simulink library "Hquad_control_LIB_LQRI"  (Simulink 7.6)
settings: Solver=ode45  StartTime=0.0  StopTime=10.0  RelTol=1e-3
values from neighbouring files (symbols this model uses):
  delay_pade_order = 0    [kostas_malakies.mat]    (also in kostas_malakies2.mat; main.m; main_last.m)
  g = 9.8065    [kostas_malakies.mat]    (also in kostas_malakies2.mat; load_PMModel.m = 9.81; main_last.m; matlab.mat)
  K_I_lqri_x = 0.330095898719    [kostas_malakies.mat]    (also in kostas_malakies2.mat)
  K_I_lqri_y = -0.330255855134    [kostas_malakies.mat]    (also in kostas_malakies2.mat)
  K_I_lqri_yaw = -0.366670548052    [kostas_malakies.mat]    (also in kostas_malakies2.mat)
  K_I_lqri_z = 0.689854163424    [kostas_malakies.mat]    (also in kostas_malakies2.mat)
  K_lqri_x = [-0.894732962063 -0.662437896475 0.0253750911961 0.0106501878726]    [kostas_malakies.mat]    (also in kostas_malakies2.mat)
  K_lqri_y = [0.897498772304 0.669088738193 0.0296050685235 0.0123545448922]    [kostas_malakies.mat]    (also in kostas_malakies2.mat)
  K_lqri_yaw = [1.88702639282 0.555643586179]    [kostas_malakies.mat]    (also in kostas_malakies2.mat)
  K_lqri_z = [-2.31070216446 -2.1452727372]    [kostas_malakies.mat]    (also in kostas_malakies2.mat)
  kalm_lqri_x =     [kostas_malakies.mat]    (also in kostas_malakies2.mat)
  kalm_lqri_y =     [kostas_malakies.mat]    (also in kostas_malakies2.mat)
  kalm_lqri_yaw =     [kostas_malakies.mat]    (also in kostas_malakies2.mat)
  kalm_lqri_z =     [kostas_malakies.mat]    (also in kostas_malakies2.mat)
  mass = 0.66    [kostas_malakies.mat]    (also in kostas_malakies2.mat; load_PMModel.m = 0.687; main_last.m)
  MAX_ANGLE = 0.261799387799    [kostas_malakies.mat]    (also in kostas_malakies2.mat; main.m; main_last.m)
  MAX_FORCE = 2    [kostas_malakies.mat]    (also in kostas_malakies2.mat; main.m; main_last.m)
  MAX_YAW_RATE = 3.14159265359    [kostas_malakies.mat]    (also in kostas_malakies2.mat; main.m; main_last.m)
  Ts = 0.02    [kostas_malakies.mat]    (also in kostas_malakies2.mat; main.m; main_last.m; matlab.mat = 0.08)
undefined symbols (not defined in the file or in its folder): DiscIntNeverNeededParam
libraries: Hquad_control_LIB_LQRI x17, simulink x9
settings Model: Creator=andi  LastModifiedBy=burrimi

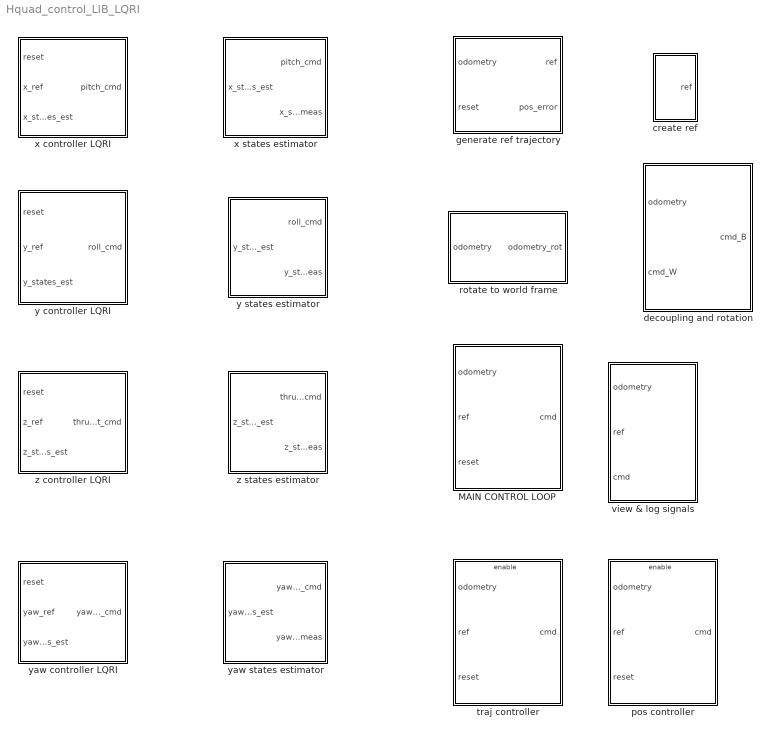
== system Hquad_control_LIB_LQRI ==
  MAIN CONTROL LOOP : Subsystem  TreatAsAtomicUnit=on
  create ref : Subsystem
  decoupling and rotation : Subsystem  Priority=3  TreatAsAtomicUnit=on
  generate ref trajectory : Subsystem
  pos controller : Subsystem
  rotate to world frame : Subsystem  Priority=1
  traj controller : Subsystem
  view & log signals : Subsystem
  "x controller LQRI  " : Subsystem
  x states estimator : Subsystem
  y controller LQRI : Subsystem
  y states estimator : Subsystem
  yaw controller LQRI : Subsystem
  yaw states estimator : Subsystem
  z controller LQRI : Subsystem
  z states estimator : Subsystem

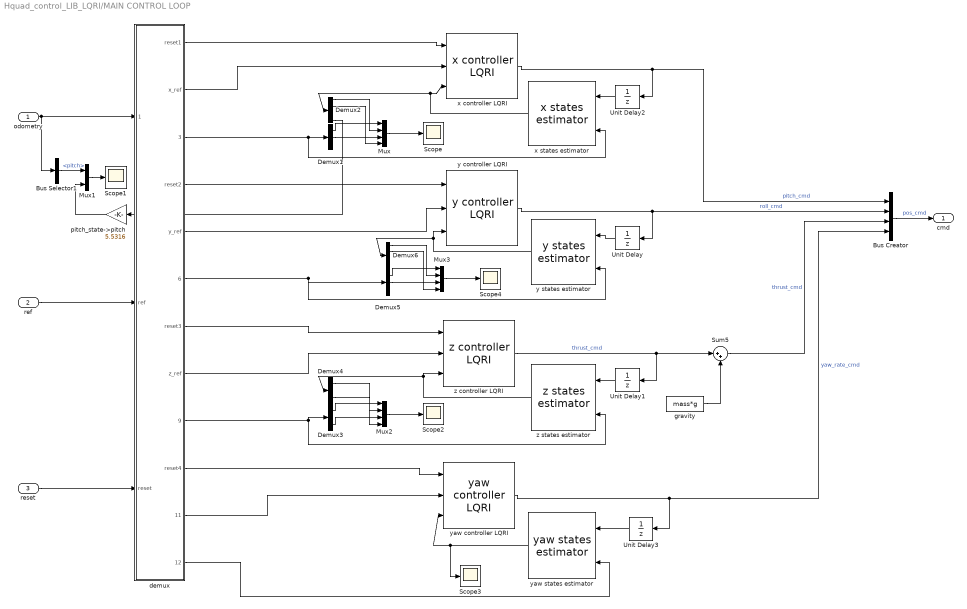
== system Hquad_control_LIB_LQRI/MAIN CONTROL LOOP ==
  odometry : Inport
  ref : Inport  Port=2
  reset : Inport  Port=3
  Bus Creator : BusCreator
  Bus Selector1 : BusSelector  OutputSignals=rpy.pitch
  Demux1 : Demux  Outputs=3
  Demux2 : Demux
  Demux3 : Demux  Outputs=2
  Demux4 : Demux  Outputs=2
  Demux5 : Demux  Outputs=3
  Demux6 : Demux
  Mux : Mux
  Mux1 : Mux  Inputs=2
  Mux2 : Mux
  Mux3 : Mux
  Scope{,1..4} (5 alike) : Scope
      Scope settings: TimeRange=8.564360869565219  YMin=-0.05  YMax=1.05  SaveName=ScopeData13
      Scope1 settings: YMin=-0.4  YMax=1.4  SaveName=ScopeData14
      Scope2 settings: YMin=-0.4  YMax=1.4  SaveName=ScopeData15
      Scope3 settings: YMin=-0.4  YMax=1.4  SaveName=ScopeData16
      Scope4 settings: TimeRange=8.564360869565219  YMin=-0.05  YMax=1.05  SaveName=ScopeData4
  Sum5 : Sum  Inputs=|++
  Unit Delay{,1..3} (4 alike) : UnitDelay  SampleTime=Ts
  demux : Subsystem
  gravity : Constant  Value=mass*g
  pitch_state->pitch : Gain  Gain=5.5316
  "x controller LQRI  " : Hquad_control_LIB_LQRI/x controller LQRI    SystemSampleTime=-1
  x states estimator : Hquad_control_LIB_LQRI/x states estimator  SystemSampleTime=-1
  y controller LQRI : Hquad_control_LIB_LQRI/y controller LQRI  SystemSampleTime=-1
  y states estimator : Hquad_control_LIB_LQRI/y states estimator  SystemSampleTime=-1
  yaw controller LQRI : Hquad_control_LIB_LQRI/yaw controller LQRI  SystemSampleTime=-1
  yaw states estimator : Hquad_control_LIB_LQRI/yaw states estimator  SystemSampleTime=-1
  z controller LQRI : Hquad_control_LIB_LQRI/z controller LQRI  SystemSampleTime=-1
  z states estimator : Hquad_control_LIB_LQRI/z states estimator  SystemSampleTime=-1
  cmd : Outport
  wires:
  demux/7(reset3) -> z controller LQRI/1
  demux/8(z_ref) -> z controller LQRI/2
  Demux4/2 -> Mux2/4
  Demux6/2 -> Mux3/4
  Demux5/2 -> Mux3/3
  Demux6/1 -> Mux3/2
  Demux5/1 -> Mux3/1
  Mux3/1 -> Scope4/1
  demux/4(reset2) -> y controller LQRI/1
  demux/5(y_ref) -> y controller LQRI/2
  gravity/1 -> Sum5/2
  yaw states estimator/1 -> Scope3/1, yaw controller LQRI/3
  z controller LQRI/1 -> Sum5/1, Unit Delay1/1  "thrust_cmd"
  Demux3/2 -> Mux2/3
  Demux4/1 -> Mux2/2
  Demux3/1 -> Mux2/1
  Mux2/1 -> Scope2/1
  pitch_state->pitch/1 -> Mux1/2
  Demux2/4 -> pitch_state->pitch/1
  Bus Selector1/1 -> Mux1/1  "<pitch>"
  Mux1/1 -> Scope1/1
  Demux2/2 -> Mux/4
  Demux1/2 -> Mux/3
  Demux2/1 -> Mux/2
  Demux1/1 -> Mux/1
  Mux/1 -> Scope/1
  z states estimator/1 -> Demux4/1, z controller LQRI/3
  y controller LQRI/1 -> Bus Creator/2, Unit Delay/1  "roll_cmd"
  "x controller LQRI  "/1 -> Bus Creator/1, Unit Delay2/1  "pitch_cmd"
  y states estimator/1 -> Demux6/1, y controller LQRI/3
  x states estimator/1 -> Demux2/1, "x controller LQRI  "/3
  demux/2(x_ref) -> "x controller LQRI  "/2
  Unit Delay/1 -> y states estimator/1
  Unit Delay1/1 -> z states estimator/1
  Unit Delay2/1 -> x states estimator/1
  demux/12(yaw_states_meas) -> yaw states estimator/2
  yaw controller LQRI/1 -> Bus Creator/4, Unit Delay3/1  "yaw_rate_cmd"
  odometry/1 -> Bus Selector1/1, demux/1(odometry)
  ref/1 -> demux/2(ref)
  reset/1 -> demux/3(reset)
  demux/1(reset1) -> "x controller LQRI  "/1
  demux/10(reset4) -> yaw controller LQRI/1
  Bus Creator/1 -> cmd/1  "pos_cmd"
  demux/3(x_states_meas) -> Demux1/1, x states estimator/2
  demux/6(y_states_meas) -> Demux5/1, y states estimator/2
  demux/9(z_states_meas) -> Demux3/1, z states estimator/2
  demux/11(yaw_ref) -> yaw controller LQRI/2
  Sum5/1 -> Bus Creator/3  "thrust_cmd"
  Unit Delay3/1 -> yaw states estimator/1

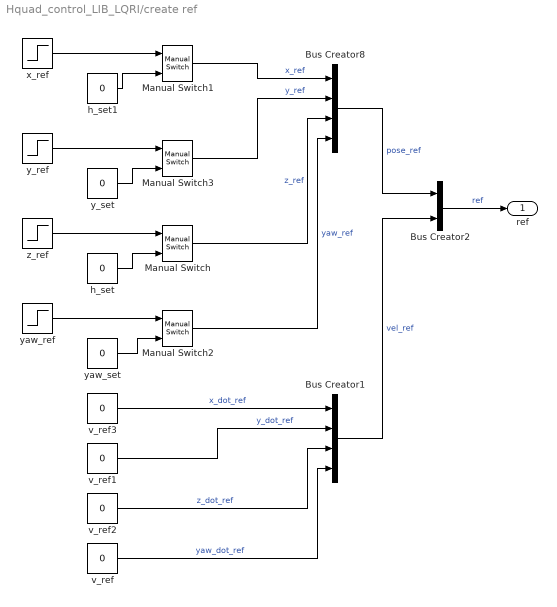
== system Hquad_control_LIB_LQRI/create ref ==
  Bus Creator1 : BusCreator
  Bus Creator2 : BusCreator  Inputs=2
  Bus Creator8 : BusCreator
  Manual Switch{,1..3} (4 alike) : simulink/Signal Routing/Manual Switch  SystemSampleTime=-1  sw=1  action=0  varsize=off
  h_set : Constant  Value=0  OutDataTypeStr=double  SampleTime=-1
  h_set1 : Constant  Value=0  OutDataTypeStr=double  SampleTime=-1
  v_ref{,1..3} (4 alike) : Constant  Value=0  OutDataTypeStr=double  SampleTime=-1
  x_ref : Step  Time=5  SampleTime=0
  y_ref : Step  Time=15  SampleTime=0
  y_set : Constant  Value=0  OutDataTypeStr=double  SampleTime=-1
  yaw_ref : Step  Time=20  After=pi  SampleTime=0
  "yaw_set  " : Constant  Value=0  OutDataTypeStr=double  SampleTime=-1
  z_ref : Step  Time=15  SampleTime=0
  ref : Outport
  wires:
  yaw_ref/1 -> Manual Switch2/1
  "yaw_set  "/1 -> Manual Switch2/2
  h_set/1 -> Manual Switch/2
  z_ref/1 -> Manual Switch/1
  y_ref/1 -> Manual Switch3/1
  y_set/1 -> Manual Switch3/2
  h_set1/1 -> Manual Switch1/2
  Bus Creator2/1 -> ref/1  "ref"
  Bus Creator8/1 -> Bus Creator2/1  "pose_ref"
  Bus Creator1/1 -> Bus Creator2/2  "vel_ref"
  Manual Switch1/1 -> Bus Creator8/1  "x_ref"
  Manual Switch3/1 -> Bus Creator8/2  "y_ref"
  Manual Switch2/1 -> Bus Creator8/4  "yaw_ref"
  Manual Switch/1 -> Bus Creator8/3  "z_ref"
  v_ref/1 -> Bus Creator1/4  "yaw_dot_ref"
  v_ref3/1 -> Bus Creator1/1  "x_dot_ref"
  v_ref1/1 -> Bus Creator1/2  "y_dot_ref"
  v_ref2/1 -> Bus Creator1/3  "z_dot_ref"
  x_ref/1 -> Manual Switch1/1

== system Hquad_control_LIB_LQRI/decoupling and rotation ==
  note: 
  odometry : Inport
  cmd_W : Inport  Port=2
  Bus Selector1 : BusSelector  OutputSignals=rpy.yaw
  Bus Selector2 : BusSelector  OutputSignals=rpy.roll,rpy.pitch
  "decoupling " : Subsystem
  rotate_to_quat_frame : Subsystem
  cmd_B : Outport
  wires:
  Bus Selector2/2 -> "decoupling "/2("pitch_meas  ")  "<pitch>"
  Bus Selector2/1 -> "decoupling "/1("roll_meas  ")  "<roll>"
  cmd_W/1 -> "decoupling "/3(cmd)
  Bus Selector1/1 -> rotate_to_quat_frame/1(yaw_meas)  "<yaw>"
  odometry/1 -> Bus Selector2/1, Bus Selector1/1
  "decoupling "/1("cmd_comp  ") -> rotate_to_quat_frame/2(cmd_comp)  "cmd_comp"
  rotate_to_quat_frame/1("cmd_rot  ") -> cmd_B/1  "roll_cmd"

== system Hquad_control_LIB_LQRI/generate ref trajectory ==
  odometry : Inport
  reset : Inport  Port=2
  Bus Creator : BusCreator
  Bus Creator1 : BusCreator
  Bus Creator2 : BusCreator  Inputs=2
  Bus Selector : BusSelector  OutputSignals=pos,vel
  Demux : Demux  Outputs=2
  Demux1 : Demux  Outputs=3
  Demux2 : Demux  Outputs=3
  Embedded MATLAB Function : Stateflow chart  TreatAsAtomicUnit=on
  Unit Delay Resettable : simulink/Additional Math & Discrete/Additional Discrete/Unit Delay Resettable  SystemSampleTime=-1  vinit=0.0  tsamp=-1
  ref : Outport
  pos_error : Outport  Port=2
  wires:
  Bus Creator2/1 -> ref/1  "ref"
  reset/1 -> Unit Delay Resettable/2
  Bus Creator1/1 -> Bus Creator2/2  "vel_ref"
  Bus Creator/1 -> Bus Creator2/1  "pose_ref"
  Demux/2 -> Bus Creator1/4  "yaw_dot_ref"
  Demux2/3 -> Bus Creator1/3  "z_dot_ref"
  Demux2/2 -> Bus Creator1/2  "y_dot_ref"
  Demux2/1 -> Bus Creator1/1  "x_dot_ref"
  Demux/1 -> Bus Creator/4  "yaw_ref"
  Demux1/3 -> Bus Creator/3  "z_ref"
  Demux1/2 -> Bus Creator/2  "y_ref"
  Demux1/1 -> Bus Creator/1  "x_ref"
  Embedded MATLAB Function/2(vel_ref) -> Demux2/1
  Embedded MATLAB Function/1(pos_ref) -> Demux1/1
  Embedded MATLAB Function/4(error) -> pos_error/1  "pos_error"
  Embedded MATLAB Function/3(yaw_ref) -> Demux/1
  Embedded MATLAB Function/5(waypoint_id_out) -> Unit Delay Resettable/1
  Unit Delay Resettable/1 -> Embedded MATLAB Function/3(waypoint_id)
  odometry/1 -> Bus Selector/1
  Bus Selector/1 -> Embedded MATLAB Function/1(pos)  "<pos>"
  Bus Selector/2 -> Embedded MATLAB Function/2(vel)  "<vel>"

== system Hquad_control_LIB_LQRI/pos controller ==
  odometry : Inport
  ref : Inport  Port=2
  reset : Inport  Port=3
  Enable : EnablePort  StatesWhenEnabling=reset
  MAIN CONTROL LOOP : Hquad_control_LIB_LQRI/MAIN CONTROL LOOP  SystemSampleTime=-1
  decoupling and rotation : Hquad_control_LIB_LQRI/decoupling and rotation  Priority=3  SystemSampleTime=-1
  rotate to world frame : Hquad_control_LIB_LQRI/rotate to world frame  Priority=1  SystemSampleTime=-1
  view & log signals : Hquad_control_LIB_LQRI/view & log signals  SystemSampleTime=-1
  cmd : Outport
  wires:
  ref/1 -> MAIN CONTROL LOOP/2, view & log signals/2
  reset/1 -> MAIN CONTROL LOOP/3
  odometry/1 -> rotate to world frame/1
  rotate to world frame/1 -> view & log signals/1, decoupling and rotation/1, MAIN CONTROL LOOP/1
  MAIN CONTROL LOOP/1 -> view & log signals/3, decoupling and rotation/2
  decoupling and rotation/1 -> cmd/1

== system Hquad_control_LIB_LQRI/rotate to world frame ==
  odometry : Inport
  Bus Creator1 : BusCreator  Inputs=3
  Bus Creator5 : BusCreator
  Bus Selector1 : BusSelector  OutputSignals=rpy.roll,rpy.pitch
  Bus Selector2 : BusSelector  OutputSignals=ang_vel
  Bus Selector3 : BusSelector  OutputSignals=rpy.yaw
  Bus Selector6 : BusSelector  OutputSignals=pos,vel
  Embedded MATLAB Function : Stateflow chart  TreatAsAtomicUnit=on
  odometry_rot : Outport
  wires:
  Bus Selector1/2 -> Embedded MATLAB Function/2(pitch)  "<pitch>"
  Bus Selector1/1 -> Embedded MATLAB Function/1(roll)  "<roll>"
  Embedded MATLAB Function/2(pitch_rot) -> Bus Creator1/2  "pitch"
  Embedded MATLAB Function/1(roll_rot) -> Bus Creator1/1  "roll"
  Bus Creator1/1 -> Bus Creator5/3  "rpy"
  Bus Selector2/1 -> Bus Creator5/4  "<ang_vel>"
  odometry/1 -> Bus Selector2/1, Bus Selector6/1, Bus Selector1/1, Bus Selector3/1
  Bus Selector3/1 -> Bus Creator1/3, Embedded MATLAB Function/3(yaw)  "<yaw>"
  Bus Creator5/1 -> odometry_rot/1  "odom"
  Bus Selector6/1 -> Bus Creator5/1  "<pos>"
  Bus Selector6/2 -> Bus Creator5/2  "<vel>"

== system Hquad_control_LIB_LQRI/traj controller ==
  odometry : Inport
  ref : Inport  Port=2
  reset : Inport  Port=3
  Enable : EnablePort  StatesWhenEnabling=reset
  MAIN CONTROL LOOP : Hquad_control_LIB_LQRI/MAIN CONTROL LOOP  SystemSampleTime=-1
  Terminator : Terminator
  decoupling and rotation : Hquad_control_LIB_LQRI/decoupling and rotation  Priority=3  SystemSampleTime=-1
  generate ref trajectory : Hquad_control_LIB_LQRI/generate ref trajectory  SystemSampleTime=-1
  rotate to world frame : Hquad_control_LIB_LQRI/rotate to world frame  Priority=1  SystemSampleTime=-1
  view & log signals : Hquad_control_LIB_LQRI/view & log signals  SystemSampleTime=-1
  cmd : Outport
  wires:
  decoupling and rotation/1 -> cmd/1
  MAIN CONTROL LOOP/1 -> decoupling and rotation/2, view & log signals/3
  rotate to world frame/1 -> MAIN CONTROL LOOP/1, decoupling and rotation/1, view & log signals/1
  odometry/1 -> rotate to world frame/1, generate ref trajectory/1
  ref/1 -> Terminator/1
  reset/1 -> MAIN CONTROL LOOP/3, generate ref trajectory/2
  generate ref trajectory/1 -> view & log signals/2, MAIN CONTROL LOOP/2

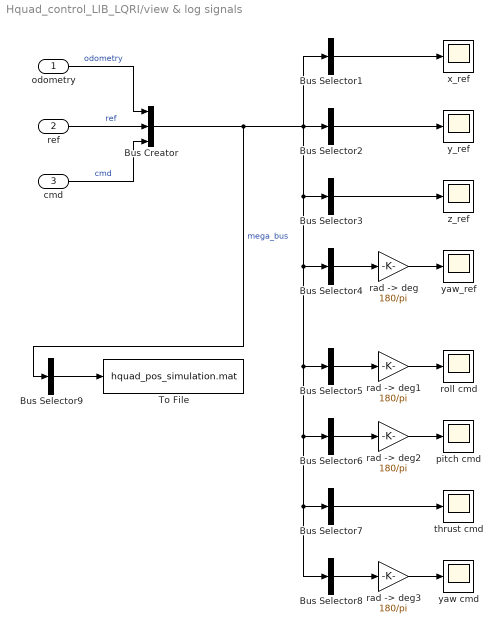
== system Hquad_control_LIB_LQRI/view & log signals ==
  odometry : Inport
  ref : Inport  Port=2
  cmd : Inport  Port=3
  Bus Creator : BusCreator  Inputs=3
  Bus Selector1 : BusSelector  OutputSignals=odometry.pos.x,odometry.vel.x_dot,ref.pose_ref.x_ref,ref.vel_ref.x_dot_ref  OutputAsBus=on
  Bus Selector2 : BusSelector  OutputSignals=odometry.pos.y,odometry.vel.y_dot,ref.pose_ref.y_ref,ref.vel_ref.y_dot_ref  OutputAsBus=on
  Bus Selector3 : BusSelector  OutputSignals=odometry.pos.z,odometry.vel.z_dot,ref.pose_ref.z_ref,ref.vel_ref.z_dot_ref  OutputAsBus=on
  Bus Selector4 : BusSelector  OutputSignals=odometry.rpy.yaw,odometry.ang_vel.ang_vel_z,ref.pose_ref.yaw_ref,ref.vel_ref.yaw_dot_ref  OutputAsBus=on
  Bus Selector5 : BusSelector  OutputSignals=odometry.rpy.roll,odometry.ang_vel.ang_vel_x,cmd.roll_cmd  OutputAsBus=on
  Bus Selector6 : BusSelector  OutputSignals=odometry.rpy.pitch,odometry.ang_vel.ang_vel_y,cmd.pitch_cmd  OutputAsBus=on
  Bus Selector7 : BusSelector  OutputSignals=odometry.pos.z,ref.pose_ref.z_ref,cmd.thrust_cmd  OutputAsBus=on
  Bus Selector8 : BusSelector  OutputSignals=odometry.rpy.yaw,odometry.ang_vel.ang_vel_z,cmd.yaw_rate_cmd  OutputAsBus=on
  Bus Selector9 : BusSelector  OutputSignals=odometry.pos.x,odometry.vel.x_dot,odometry.rpy.pitch,ref.pose_ref.x_ref,cmd.pitch_cmd,odometry.pos.y,odometry.vel.y_dot,odometry.rpy.roll,ref.pose_ref.y_ref,cmd.roll_cmd,odometry.pos.z,odometry.vel.z_dot,ref.pose_ref.z_ref,cmd.thrust_cmd,odometry.rpy.yaw,odometry.ang_vel.ang_vel_z,ref.pose_ref.yaw_ref,cmd.yaw_rate_cmd  OutputAsBus=on
  To File : ToFile  Filename=hquad_pos_simulation.mat  MatrixName=hquad_pos_simulation
  pitch cmd : Scope
      settings: YMin=-15  YMax=15  SaveName=ScopeData2
  rad -> deg{,1..3} (4 alike) : Gain  Gain=180/pi
  roll cmd : Scope
      settings: YMin=-100  YMax=100
  thrust cmd : Scope
      settings: YMin=-3  YMax=3  SaveName=ScopeData11
  x_ref : Scope
      settings: TimeRange=40  YMin=-1.5  YMax=1.5  SaveName=ScopeData3
  y_ref : Scope
      settings: TimeRange=40  YMin=-1.5  YMax=1.5
  yaw cmd : Scope
      settings: YMin=-60  YMax=-0  SaveName=ScopeData10
  yaw_ref : Scope
      settings: TimeRange=39.996  YMin=0  YMax=3250  SaveName=ScopeData8
  z_ref : Scope
      settings: YMin=-0.05  YMax=1.05  SaveName=ScopeData5
  wires:
  Bus Selector8/1 -> "rad -> deg3"/1
  Bus Selector6/1 -> "rad -> deg2"/1
  Bus Selector5/1 -> "rad -> deg1"/1
  Bus Selector7/1 -> thrust cmd/1
  Bus Selector4/1 -> "rad -> deg"/1
  Bus Selector3/1 -> z_ref/1
  Bus Selector2/1 -> y_ref/1
  Bus Selector1/1 -> x_ref/1
  Bus Creator/1 -> Bus Selector8/1, Bus Selector7/1, Bus Selector6/1, Bus Selector5/1, Bus Selector4/1, Bus Selector3/1, Bus Selector2/1, Bus Selector1/1, Bus Selector9/1  "mega_bus"
  cmd/1 -> Bus Creator/3  "cmd"
  ref/1 -> Bus Creator/2  "ref"
  odometry/1 -> Bus Creator/1  "odometry"
  "rad -> deg3"/1 -> yaw cmd/1
  "rad -> deg2"/1 -> pitch cmd/1
  "rad -> deg1"/1 -> roll cmd/1
  "rad -> deg"/1 -> yaw_ref/1
  Bus Selector9/1 -> To File/1

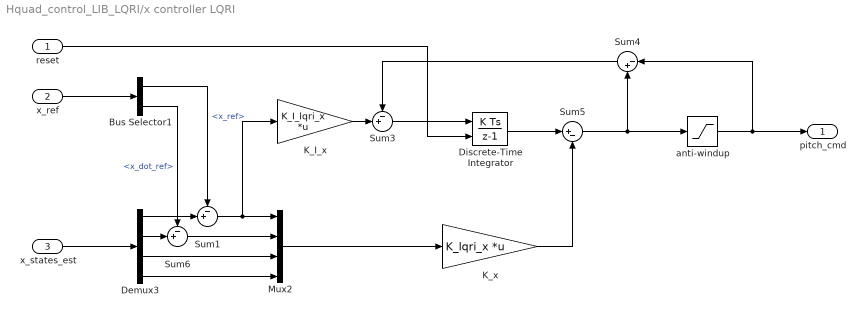
== system Hquad_control_LIB_LQRI/x controller LQRI   ==
  reset : Inport  PortDimensions=1
  "x_ref  " : Inport  Port=2  PortDimensions=2
  "x_states_est  " : Inport  Port=3
  Bus Selector1 : BusSelector  OutputSignals=x_ref,x_dot_ref
  Demux3 : Demux
  Discrete-Time Integrator : DiscreteIntegrator  ExternalReset=rising  SampleTime=Ts  ICPrevOutput=DiscIntNeverNeededParam  ICPrevScaledInput=DiscIntNeverNeededParam
  K_I_x : Gain  Gain=K_I_lqri_x  Multiplication=Matrix(K*u)  OutDataTypeStr=single
  K_x : Gain  Gain=K_lqri_x  Multiplication=Matrix(K*u)
  Mux2 : Mux
  Sum1 : Sum  Inputs=-+|
  Sum3 : Sum  Inputs=-+|
  Sum4 : Sum  Inputs=|-+
  Sum5 : Sum  Inputs=|+-
  Sum6 : Sum  Inputs=-+|
  anti-windup : Saturate  UpperLimit=MAX_ANGLE  LowerLimit=-MAX_ANGLE
  "pitch_cmd   " : Outport  PortDimensions=1
  wires:
  Demux3/2 -> Sum6/2
  Bus Selector1/2 -> Sum6/1  "<x_dot_ref>"
  Bus Selector1/1 -> Sum1/1  "<x_ref>"
  Sum6/1 -> Mux2/2
  "x_ref  "/1 -> Bus Selector1/1
  Sum3/1 -> Discrete-Time Integrator/1
  Sum4/1 -> Sum3/1
  Discrete-Time Integrator/1 -> Sum5/1
  K_x/1 -> Sum5/2
  anti-windup/1 -> "pitch_cmd   "/1, Sum4/1
  reset/1 -> Discrete-Time Integrator/2
  "x_states_est  "/1 -> Demux3/1
  Mux2/1 -> K_x/1
  Demux3/1 -> Sum1/2
  Sum1/1 -> Mux2/1, K_I_x/1
  Demux3/3 -> Mux2/3
  Demux3/4 -> Mux2/4
  K_I_x/1 -> Sum3/2
  Sum5/1 -> anti-windup/1, Sum4/2

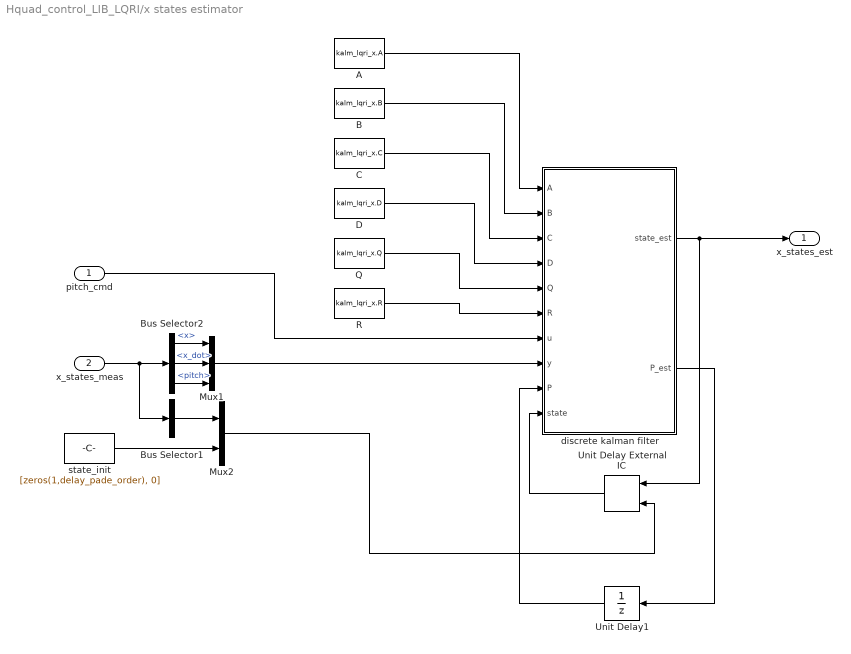
== system Hquad_control_LIB_LQRI/x states estimator ==
  pitch_cmd : Inport  PortDimensions=1
  x_states_meas : Inport  Port=2  PortDimensions=3
  A : Constant  Value=kalm_lqri_x.A
  B : Constant  Value=kalm_lqri_x.B
  Bus Selector1 : BusSelector  OutputSignals=x,x_dot,pitch  OutputAsBus=on
  Bus Selector2 : BusSelector  OutputSignals=x,x_dot,pitch
  C : Constant  Value=kalm_lqri_x.C
  D : Constant  Value=kalm_lqri_x.D
  Mux1 : Mux  Inputs=3
  Mux2 : Mux  Inputs=2
  Q : Constant  Value=kalm_lqri_x.Q
  R : Constant  Value=kalm_lqri_x.R
  Unit Delay External IC : simulink/Additional Math & Discrete/Additional Discrete/Unit Delay External IC  SystemSampleTime=-1  tsamp=-1
  Unit Delay1 : UnitDelay  X0=kalm_lqri_x.Z  SampleTime=Ts
  discrete kalman filter : Stateflow chart  TreatAsAtomicUnit=on
  state_init : Constant  Value=[zeros(1,delay_pade_order), 0]
  x_states_est : Outport  PortDimensions=4+delay_pade_order
  wires:
  x_states_meas/1 -> Bus Selector1/1, Bus Selector2/1
  state_init/1 -> Mux2/2
  Bus Selector1/1 -> Mux2/1
  A/1 -> discrete kalman filter/1(A)
  B/1 -> discrete kalman filter/2(B)
  C/1 -> discrete kalman filter/3(C)
  D/1 -> discrete kalman filter/4(D)
  discrete kalman filter/1(state_est) -> x_states_est/1, Unit Delay External IC/1
  Unit Delay External IC/1 -> discrete kalman filter/10(state)
  discrete kalman filter/2(P_est) -> Unit Delay1/1
  Unit Delay1/1 -> discrete kalman filter/9(P)
  Mux2/1 -> Unit Delay External IC/2
  pitch_cmd/1 -> discrete kalman filter/7(u)
  Bus Selector2/1 -> Mux1/1  "<x>"
  Bus Selector2/2 -> Mux1/2  "<x_dot>"
  Bus Selector2/3 -> Mux1/3  "<pitch>"
  Mux1/1 -> discrete kalman filter/8(y)
  Q/1 -> discrete kalman filter/5(Q)
  R/1 -> discrete kalman filter/6(R)

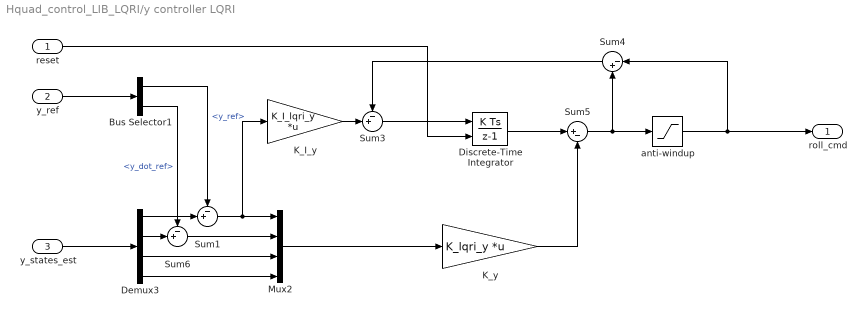
== system Hquad_control_LIB_LQRI/y controller LQRI ==
  reset : Inport  PortDimensions=1
  "y_ref  " : Inport  Port=2  PortDimensions=2
  "y_states_est  " : Inport  Port=3
  Bus Selector1 : BusSelector  OutputSignals=y_ref,y_dot_ref
  Demux3 : Demux
  Discrete-Time Integrator : DiscreteIntegrator  ExternalReset=rising  SampleTime=Ts  ICPrevOutput=DiscIntNeverNeededParam  ICPrevScaledInput=DiscIntNeverNeededParam
  K_I_y : Gain  Gain=K_I_lqri_y  Multiplication=Matrix(K*u)  OutDataTypeStr=single
  K_y : Gain  Gain=K_lqri_y  Multiplication=Matrix(K*u)
  Mux2 : Mux
  Sum1 : Sum  Inputs=-+|
  Sum3 : Sum  Inputs=-+|
  Sum4 : Sum  Inputs=|-+
  Sum5 : Sum  Inputs=|+-
  Sum6 : Sum  Inputs=-+|
  anti-windup : Saturate  UpperLimit=MAX_ANGLE  LowerLimit=-MAX_ANGLE
  "roll_cmd   " : Outport  PortDimensions=1
  wires:
  Demux3/2 -> Sum6/2
  Bus Selector1/2 -> Sum6/1  "<y_dot_ref>"
  Bus Selector1/1 -> Sum1/1  "<y_ref>"
  Sum6/1 -> Mux2/2
  "y_ref  "/1 -> Bus Selector1/1
  Sum3/1 -> Discrete-Time Integrator/1
  Sum4/1 -> Sum3/1
  Discrete-Time Integrator/1 -> Sum5/1
  K_y/1 -> Sum5/2
  anti-windup/1 -> "roll_cmd   "/1, Sum4/1
  reset/1 -> Discrete-Time Integrator/2
  "y_states_est  "/1 -> Demux3/1
  Mux2/1 -> K_y/1
  Demux3/1 -> Sum1/2
  Sum1/1 -> Mux2/1, K_I_y/1
  Demux3/3 -> Mux2/3
  Demux3/4 -> Mux2/4
  K_I_y/1 -> Sum3/2
  Sum5/1 -> anti-windup/1, Sum4/2

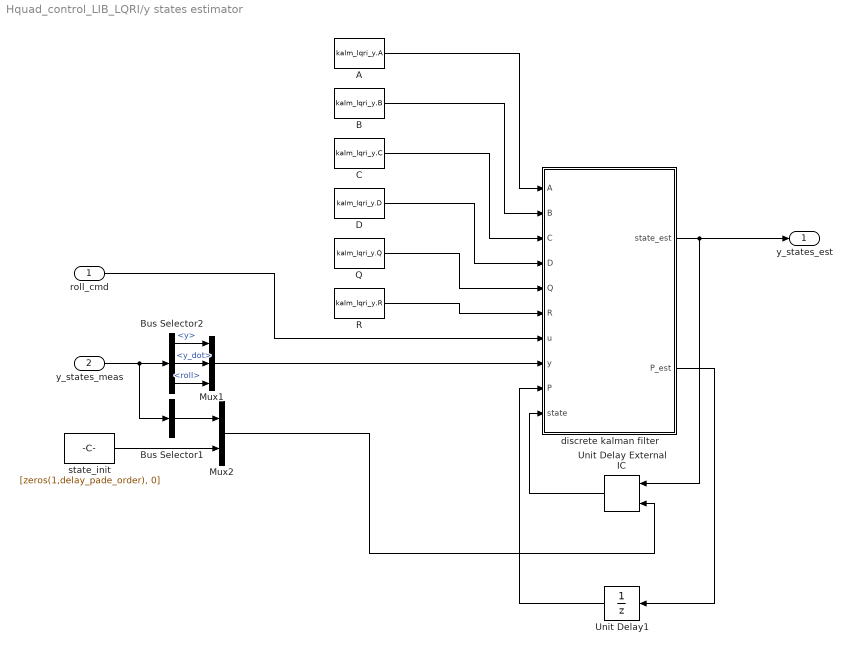
== system Hquad_control_LIB_LQRI/y states estimator ==
  roll_cmd : Inport  PortDimensions=1
  y_states_meas : Inport  Port=2  PortDimensions=3
  A : Constant  Value=kalm_lqri_y.A
  B : Constant  Value=kalm_lqri_y.B
  Bus Selector1 : BusSelector  OutputSignals=y,y_dot,roll  OutputAsBus=on
  Bus Selector2 : BusSelector  OutputSignals=y,y_dot,roll
  C : Constant  Value=kalm_lqri_y.C
  D : Constant  Value=kalm_lqri_y.D
  Mux1 : Mux  Inputs=3
  Mux2 : Mux  Inputs=2
  Q : Constant  Value=kalm_lqri_y.Q
  R : Constant  Value=kalm_lqri_y.R
  Unit Delay External IC : simulink/Additional Math & Discrete/Additional Discrete/Unit Delay External IC  SystemSampleTime=-1  tsamp=-1
  Unit Delay1 : UnitDelay  X0=kalm_lqri_y.Z  SampleTime=Ts
  discrete kalman filter : Stateflow chart  TreatAsAtomicUnit=on
  state_init : Constant  Value=[zeros(1,delay_pade_order), 0]
  y_states_est : Outport  PortDimensions=4+delay_pade_order
  wires:
  y_states_meas/1 -> Bus Selector1/1, Bus Selector2/1
  state_init/1 -> Mux2/2
  Bus Selector1/1 -> Mux2/1
  A/1 -> discrete kalman filter/1(A)
  B/1 -> discrete kalman filter/2(B)
  C/1 -> discrete kalman filter/3(C)
  D/1 -> discrete kalman filter/4(D)
  discrete kalman filter/1(state_est) -> y_states_est/1, Unit Delay External IC/1
  Unit Delay External IC/1 -> discrete kalman filter/10(state)
  discrete kalman filter/2(P_est) -> Unit Delay1/1
  Unit Delay1/1 -> discrete kalman filter/9(P)
  Mux2/1 -> Unit Delay External IC/2
  roll_cmd/1 -> discrete kalman filter/7(u)
  Bus Selector2/1 -> Mux1/1  "<y>"
  Bus Selector2/2 -> Mux1/2  "<y_dot>"
  Bus Selector2/3 -> Mux1/3  "<roll>"
  Mux1/1 -> discrete kalman filter/8(y)
  Q/1 -> discrete kalman filter/5(Q)
  R/1 -> discrete kalman filter/6(R)

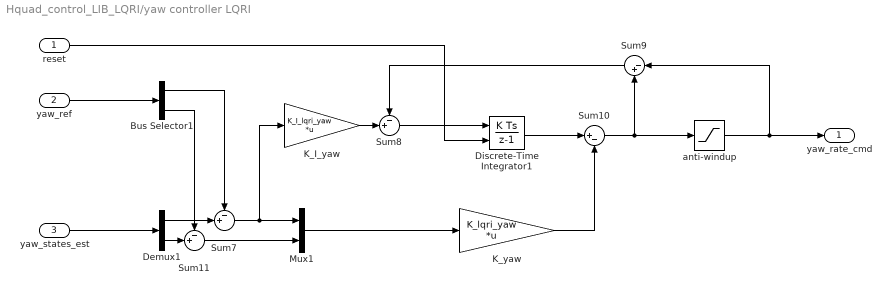
== system Hquad_control_LIB_LQRI/yaw controller LQRI ==
  reset : Inport  PortDimensions=1
  "yaw_ref  " : Inport  Port=2  PortDimensions=2
  "yaw_states_est  " : Inport  Port=3
  Bus Selector1 : BusSelector  OutputSignals=yaw_ref,yaw_dot_ref
  Demux1 : Demux  Outputs=2
  Discrete-Time Integrator1 : DiscreteIntegrator  ExternalReset=rising  SampleTime=Ts  ICPrevOutput=DiscIntNeverNeededParam  ICPrevScaledInput=DiscIntNeverNeededParam
  K_I_yaw : Gain  Gain=K_I_lqri_yaw  Multiplication=Matrix(K*u)  OutDataTypeStr=single
  K_yaw : Gain  Gain=K_lqri_yaw  Multiplication=Matrix(K*u)
  Mux1 : Mux  Inputs=2
  Sum10 : Sum  Inputs=|+-
  Sum11 : Sum  Inputs=-+|
  Sum7 : Sum  Inputs=-+|
  Sum8 : Sum  Inputs=-+|
  Sum9 : Sum  Inputs=|-+
  anti-windup : Saturate  UpperLimit=MAX_YAW_RATE  LowerLimit=-MAX_YAW_RATE
  "yaw_rate_cmd  " : Outport  PortDimensions=1
  wires:
  Demux1/2 -> Sum11/2
  Bus Selector1/2 -> Sum11/1
  Bus Selector1/1 -> Sum7/1
  Sum11/1 -> Mux1/2
  Sum8/1 -> Discrete-Time Integrator1/1
  Sum9/1 -> Sum8/1
  Discrete-Time Integrator1/1 -> Sum10/1
  K_yaw/1 -> Sum10/2
  reset/1 -> Discrete-Time Integrator1/2
  "yaw_states_est  "/1 -> Demux1/1
  Mux1/1 -> K_yaw/1
  Demux1/1 -> Sum7/2
  Sum7/1 -> Mux1/1, K_I_yaw/1
  K_I_yaw/1 -> Sum8/2
  Sum10/1 -> anti-windup/1, Sum9/2
  "yaw_ref  "/1 -> Bus Selector1/1
  anti-windup/1 -> "yaw_rate_cmd  "/1, Sum9/1

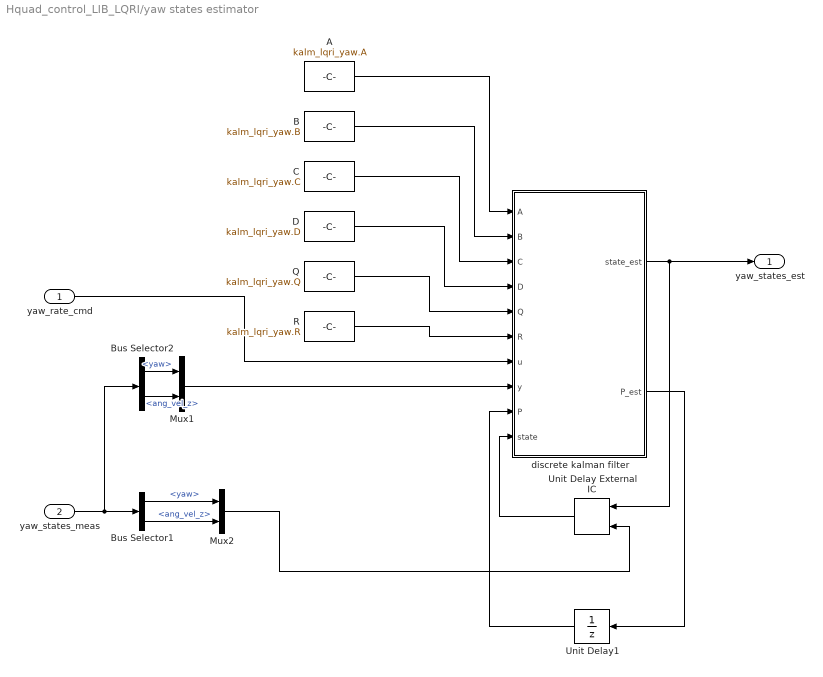
== system Hquad_control_LIB_LQRI/yaw states estimator ==
  yaw_rate_cmd : Inport  PortDimensions=1
  yaw_states_meas : Inport  Port=2  PortDimensions=2
  A : Constant  Value=kalm_lqri_yaw.A
  B : Constant  Value=kalm_lqri_yaw.B
  Bus Selector1 : BusSelector  OutputSignals=yaw,ang_vel_z
  Bus Selector2 : BusSelector  OutputSignals=yaw,ang_vel_z
  C : Constant  Value=kalm_lqri_yaw.C
  D : Constant  Value=kalm_lqri_yaw.D
  Mux1 : Mux  Inputs=2
  Mux2 : Mux  Inputs=2
  Q : Constant  Value=kalm_lqri_yaw.Q
  R : Constant  Value=kalm_lqri_yaw.R
  Unit Delay External IC : simulink/Additional Math & Discrete/Additional Discrete/Unit Delay External IC  SystemSampleTime=-1  tsamp=-1
  Unit Delay1 : UnitDelay  X0=kalm_lqri_yaw.Z  SampleTime=Ts
  discrete kalman filter : Stateflow chart  TreatAsAtomicUnit=on
  yaw_states_est : Outport  PortDimensions=2+delay_pade_order
  wires:
  Mux2/1 -> Unit Delay External IC/2
  Bus Selector1/2 -> Mux2/2  "<ang_vel_z>"
  Bus Selector1/1 -> Mux2/1  "<yaw>"
  R/1 -> discrete kalman filter/6(R)
  Q/1 -> discrete kalman filter/5(Q)
  Mux1/1 -> discrete kalman filter/8(y)
  Bus Selector2/2 -> Mux1/2  "<ang_vel_z>"
  Bus Selector2/1 -> Mux1/1  "<yaw>"
  yaw_rate_cmd/1 -> discrete kalman filter/7(u)
  Unit Delay1/1 -> discrete kalman filter/9(P)
  discrete kalman filter/2(P_est) -> Unit Delay1/1
  Unit Delay External IC/1 -> discrete kalman filter/10(state)
  discrete kalman filter/1(state_est) -> Unit Delay External IC/1, yaw_states_est/1
  D/1 -> discrete kalman filter/4(D)
  C/1 -> discrete kalman filter/3(C)
  B/1 -> discrete kalman filter/2(B)
  A/1 -> discrete kalman filter/1(A)
  yaw_states_meas/1 -> Bus Selector1/1, Bus Selector2/1

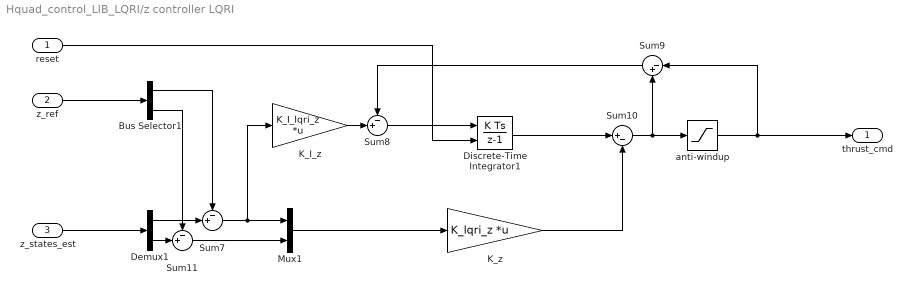
== system Hquad_control_LIB_LQRI/z controller LQRI ==
  reset : Inport  PortDimensions=1
  "z_ref  " : Inport  Port=2  PortDimensions=2
  "z_states_est  " : Inport  Port=3
  Bus Selector1 : BusSelector  OutputSignals=z_ref,z_dot_ref
  Demux1 : Demux  Outputs=2
  Discrete-Time Integrator1 : DiscreteIntegrator  ExternalReset=rising  SampleTime=Ts  ICPrevOutput=DiscIntNeverNeededParam  ICPrevScaledInput=DiscIntNeverNeededParam
  K_I_z : Gain  Gain=K_I_lqri_z  Multiplication=Matrix(K*u)  OutDataTypeStr=single
  K_z : Gain  Gain=K_lqri_z  Multiplication=Matrix(K*u)
  Mux1 : Mux  Inputs=2
  Sum10 : Sum  Inputs=|+-
  Sum11 : Sum  Inputs=-+|
  Sum7 : Sum  Inputs=-+|
  Sum8 : Sum  Inputs=-+|
  Sum9 : Sum  Inputs=|-+
  anti-windup : Saturate  UpperLimit=MAX_FORCE  LowerLimit=-MAX_FORCE
  "thrust_cmd  " : Outport  PortDimensions=1
  wires:
  Demux1/2 -> Sum11/2
  Bus Selector1/2 -> Sum11/1
  Bus Selector1/1 -> Sum7/1
  Sum11/1 -> Mux1/2
  Sum8/1 -> Discrete-Time Integrator1/1
  Sum9/1 -> Sum8/1
  Discrete-Time Integrator1/1 -> Sum10/1
  K_z/1 -> Sum10/2
  reset/1 -> Discrete-Time Integrator1/2
  "z_states_est  "/1 -> Demux1/1
  Mux1/1 -> K_z/1
  Demux1/1 -> Sum7/2
  Sum7/1 -> Mux1/1, K_I_z/1
  K_I_z/1 -> Sum8/2
  Sum10/1 -> anti-windup/1, Sum9/2
  "z_ref  "/1 -> Bus Selector1/1
  anti-windup/1 -> "thrust_cmd  "/1, Sum9/1

== system Hquad_control_LIB_LQRI/z states estimator ==
  thrust_cmd : Inport  PortDimensions=1
  z_states_meas : Inport  Port=2  PortDimensions=2
  A : Constant  Value=kalm_lqri_z.A
  B : Constant  Value=kalm_lqri_z.B
  Bus Selector1 : BusSelector  OutputSignals=z,z_dot
  Bus Selector2 : BusSelector  OutputSignals=z,z_dot
  C : Constant  Value=kalm_lqri_z.C
  D : Constant  Value=kalm_lqri_z.D
  Mux1 : Mux  Inputs=2
  Mux2 : Mux  Inputs=2
  Q : Constant  Value=kalm_lqri_z.Q
  R : Constant  Value=kalm_lqri_z.R
  Unit Delay External IC : simulink/Additional Math & Discrete/Additional Discrete/Unit Delay External IC  SystemSampleTime=-1  tsamp=-1
  Unit Delay1 : UnitDelay  X0=kalm_lqri_z.Z  SampleTime=Ts
  discrete kalman filter : Stateflow chart  TreatAsAtomicUnit=on
  z_states_est : Outport  PortDimensions=2+delay_pade_order
  wires:
  Mux2/1 -> Unit Delay External IC/2
  Bus Selector1/2 -> Mux2/2  "<z_dot>"
  Bus Selector1/1 -> Mux2/1  "<z>"
  R/1 -> discrete kalman filter/6(R)
  Q/1 -> discrete kalman filter/5(Q)
  Mux1/1 -> discrete kalman filter/8(y)
  Bus Selector2/2 -> Mux1/2  "<z_dot>"
  Bus Selector2/1 -> Mux1/1  "<z>"
  thrust_cmd/1 -> discrete kalman filter/7(u)
  Unit Delay1/1 -> discrete kalman filter/9(P)
  discrete kalman filter/2(P_est) -> Unit Delay1/1
  Unit Delay External IC/1 -> discrete kalman filter/10(state)
  discrete kalman filter/1(state_est) -> z_states_est/1, Unit Delay External IC/1
  D/1 -> discrete kalman filter/4(D)
  C/1 -> discrete kalman filter/3(C)
  B/1 -> discrete kalman filter/2(B)
  A/1 -> discrete kalman filter/1(A)
  z_states_meas/1 -> Bus Selector2/1, Bus Selector1/1

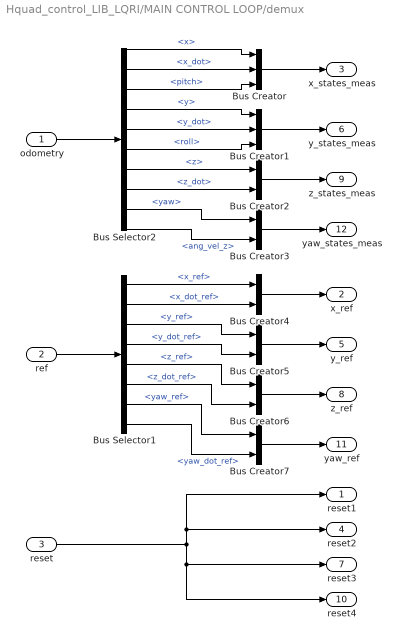
== system Hquad_control_LIB_LQRI/MAIN CONTROL LOOP/demux ==
  odometry : Inport
  ref : Inport  Port=2
  reset : Inport  Port=3
  Bus Creator : BusCreator  Inputs=3
  Bus Creator1 : BusCreator  Inputs=3
  Bus Creator{2..7} (6 alike) : BusCreator  Inputs=2
  Bus Selector1 : BusSelector  OutputSignals=pose_ref.x_ref,vel_ref.x_dot_ref,pose_ref.y_ref,vel_ref.y_dot_ref,pose_ref.z_ref,vel_ref.z_dot_ref,pose_ref.yaw_ref,vel_ref.yaw_dot_ref
  Bus Selector2 : BusSelector  OutputSignals=pos.x,vel.x_dot,rpy.pitch,pos.y,vel.y_dot,rpy.roll,pos.z,vel.z_dot,rpy.yaw,ang_vel.ang_vel_z
  reset1 : Outport
  x_ref : Outport  Port=2  PortDimensions=2
  x_states_meas : Outport  Port=3  PortDimensions=3
  reset2 : Outport  Port=4
  y_ref : Outport  Port=5  PortDimensions=2
  y_states_meas : Outport  Port=6  PortDimensions=3
  reset3 : Outport  Port=7
  z_ref : Outport  Port=8  PortDimensions=2
  z_states_meas : Outport  Port=9  PortDimensions=2
  reset4 : Outport  Port=10
  yaw_ref : Outport  Port=11  PortDimensions=2
  yaw_states_meas : Outport  Port=12  PortDimensions=2
  wires:
  Bus Selector2/6 -> Bus Creator1/3  "<roll>"
  Bus Selector2/3 -> Bus Creator/3  "<pitch>"
  odometry/1 -> Bus Selector2/1
  Bus Creator/1 -> x_states_meas/1
  Bus Selector2/1 -> Bus Creator/1  "<x>"
  Bus Selector2/2 -> Bus Creator/2  "<x_dot>"
  Bus Selector2/4 -> Bus Creator1/1  "<y>"
  Bus Selector2/5 -> Bus Creator1/2  "<y_dot>"
  Bus Creator1/1 -> y_states_meas/1
  Bus Selector2/7 -> Bus Creator2/1  "<z>"
  Bus Selector2/8 -> Bus Creator2/2  "<z_dot>"
  Bus Selector2/9 -> Bus Creator3/1  "<yaw>"
  Bus Selector2/10 -> Bus Creator3/2  "<ang_vel_z>"
  Bus Creator2/1 -> z_states_meas/1
  Bus Creator3/1 -> yaw_states_meas/1
  ref/1 -> Bus Selector1/1
  Bus Selector1/1 -> Bus Creator4/1  "<x_ref>"
  Bus Creator7/1 -> yaw_ref/1
  Bus Creator6/1 -> z_ref/1
  Bus Creator5/1 -> y_ref/1
  Bus Creator4/1 -> x_ref/1
  Bus Selector1/2 -> Bus Creator4/2  "<x_dot_ref>"
  Bus Selector1/3 -> Bus Creator5/1  "<y_ref>"
  Bus Selector1/4 -> Bus Creator5/2  "<y_dot_ref>"
  Bus Selector1/5 -> Bus Creator6/1  "<z_ref>"
  Bus Selector1/6 -> Bus Creator6/2  "<z_dot_ref>"
  Bus Selector1/7 -> Bus Creator7/1  "<yaw_ref>"
  Bus Selector1/8 -> Bus Creator7/2  "<yaw_dot_ref>"
  reset/1 -> reset3/1, reset4/1, reset2/1, reset1/1

== system Hquad_control_LIB_LQRI/decoupling and rotation/decoupling  ==
  "roll_meas  " : Inport  PortDimensions=1
  "pitch_meas  " : Inport  Port=2  PortDimensions=1
  cmd : Inport  Port=3
  Bus Creator : BusCreator
  Bus Selector3 : BusSelector  OutputSignals=pitch_cmd,roll_cmd,thrust_cmd,yaw_rate_cmd
  Embedded MATLAB Function : Stateflow chart  TreatAsAtomicUnit=on
  g : Constant  Value=g
  mass : Constant  Value=mass
  "cmd_comp  " : Outport
  wires:
  "roll_meas  "/1 -> Embedded MATLAB Function/2(roll_meas)
  "pitch_meas  "/1 -> Embedded MATLAB Function/1(pitch_meas)
  cmd/1 -> Bus Selector3/1
  Bus Selector3/4 -> Bus Creator/4  "<yaw_rate_cmd>"
  Bus Creator/1 -> "cmd_comp  "/1
  Embedded MATLAB Function/3(thrust_comp) -> Bus Creator/3  "thrust_cmd"
  Embedded MATLAB Function/2(roll_cmd_comp) -> Bus Creator/2  "roll_cmd"
  Embedded MATLAB Function/1(pitch_cmd_comp) -> Bus Creator/1  "pitch_cmd"
  Bus Selector3/1 -> Embedded MATLAB Function/3(pitch_cmd)  "<pitch_cmd>"
  Bus Selector3/2 -> Embedded MATLAB Function/4(roll_cmd)  "<roll_cmd>"
  Bus Selector3/3 -> Embedded MATLAB Function/5(thrust)  "<thrust_cmd>"
  mass/1 -> Embedded MATLAB Function/6(m)
  g/1 -> Embedded MATLAB Function/7(g)

== system Hquad_control_LIB_LQRI/decoupling and rotation/rotate_to_quat_frame ==
  yaw_meas : Inport
  cmd_comp : Inport  Port=2
  Bus Creator2 : BusCreator
  Bus Selector3 : BusSelector  OutputSignals=pitch_cmd,roll_cmd
  Bus Selector4 : BusSelector  OutputSignals=thrust_cmd,yaw_rate_cmd
  Embedded MATLAB Function : Stateflow chart  TreatAsAtomicUnit=on
  "cmd_rot  " : Outport
  wires:
  yaw_meas/1 -> Embedded MATLAB Function/1(yaw)
  Bus Creator2/1 -> "cmd_rot  "/1
  Bus Selector3/2 -> Embedded MATLAB Function/3(roll_cmd)  "<roll_cmd>"
  Bus Selector3/1 -> Embedded MATLAB Function/2(pitch_cmd)  "<pitch_cmd>"
  cmd_comp/1 -> Bus Selector3/1, Bus Selector4/1
  Embedded MATLAB Function/1(pitch_rot) -> Bus Creator2/1  "pitch_cmd"
  Embedded MATLAB Function/2(roll_rot) -> Bus Creator2/2  "roll_cmd"
  Bus Selector4/1 -> Bus Creator2/3  "<thrust_cmd>"
  Bus Selector4/2 -> Bus Creator2/4  "<yaw_rate_cmd>"

== matlab function rotate to world frame/Embedded MATLAB Function ==
  data: roll input double; pitch input double; roll_rot output double; yaw input double; pitch_rot output double
function [roll_rot,pitch_rot] = fcn(roll,pitch,yaw)
%#eml


sin_yaw=sin(yaw);
cos_yaw=cos(yaw);

R=[cos_yaw, sin_yaw; -sin_yaw, cos_yaw];

temp=R*[pitch;roll];
pitch_rot=temp(1);
roll_rot=temp(2);

== matlab function generate ref trajectory/Embedded MATLAB Function ==
  data: pos input double; pos_ref output double; vel input double; vel_ref output double; yaw_ref output double; error output double; waypoint_id input double; waypoint_id_out output double
function [pos_ref,vel_ref,yaw_ref,error,waypoint_id_out] = fcn(pos,vel,waypoint_id)
%#eml

speed=0.5;
yaw=0;

% set how fast the quadrokopter flies to first waypoint
speed_init=0.5;

% waypoints=[0,0,-1;
%         -0.5,-1,-1;
%         0.5,-0.5,-1;
%         -0.5,-0.5,-1;
%         0.5,-1,-1;
%         0,0,-1];

waypoints = [0, 0, -1, yaw, speed;
    0, -1, -1, yaw, speed;
    1, -1, -1, yaw, speed;
    1, 0, -1, yaw, speed;
    0, 0, -1, yaw, speed;
    0, -1, -1, yaw, speed;
    1, -1, -1, yaw, speed;
    1, 0, -1, yaw, speed;
    0, 0, -1, yaw, speed;
    ];





num_waypoints=size(waypoints,1);
    


%i=dsearchn(waypoints,Pos);
% d=(waypoints(:,1)-Pos(1)).^2+(waypoints(:,2)-Pos(2)).^2+(waypoints(:,3)-Pos(3)).^2
% [V,i]=min(d);
% 
% if waypoint_id~=num_waypoints && waypoint_id~=1
%     if norm(waypoints(waypoint_id-1,:)-Pos)>norm(waypoints(waypoint_id+1,:)-Pos)
%         waypoint_id=waypoint_id+1;
%     end
% end


if waypoint_id~=num_waypoints
    if waypoint_id~=0
        P1=waypoints(waypoint_id,1:3)';
        yaw1=waypoints(waypoint_id,4);
        speed=waypoints(waypoint_id,5);
    else
        P1=pos;
        % set yaw ref to ref of first waypoint
        yaw1=waypoints(1,4);
        speed=speed_init;
    end
%     P1=waypoints(waypoint_id,:)';
    P2=waypoints(waypoint_id+1,1:3)';
    yaw2=waypoints(waypoint_id+1,4);
    
    %derive vector between two waypoints
    v=(P2-P1);
    if norm(v)==0   %if 2 waypoint are equal just skip to next waypoint
        waypoint_id=waypoint_id+1;
        pos_ref=pos;
        yaw_ref=[yaw1;0];
        vel_ref=[0,0,0]';
    else
        t=(pos-P1)'*v/(v'*v);
        pos_ref=P1+t*v;
        yaw_ref=[yaw1+t*(yaw2-yaw1);0];
        % set reference velocity
        vel_ref=v/norm(v)*speed;

        % fly slower depending on the distance error from the reference
        dist_error=norm(pos_ref-pos);
        vel_ref=vel_ref*(1-dist_error*1/0.3);
        
        % set next waypoint if close enough
        if norm(pos_ref-P2)<0.05 || t>1
            waypoint_id=waypoint_id+1;
        end
    end
else %stay at the last waypoint
    pos_ref=waypoints(waypoint_id,1:3)';
    yaw_ref=[waypoints(waypoint_id,4); 0];
    vel_ref=[0,0,0]';
end

error=[norm(pos_ref-pos);norm(vel_ref-vel)];


waypoint_id_out=waypoint_id;

== matlab function x states estimator/discrete kalman filter ==
  data: A input double; B input double; state_est output double; C input double; D input double; Q input double; R input double; u input double; y input double; P input double; state input double; P_est output double
function [state_est,P_est]  = fcn(A,B,C,D,Q,R, u, y, P, state)
%#eml

% Kalman filter according to Welch & Bishop, An Introduction to the Kalman
% Filter

n=size(A,1);

% Time update
x_=A*state+B*u;
P_=A*P*A'+Q;
  
% Measurement update
K=P_*C'*(C*P_*C'+R)^-1;
state_est=x_+K*(y-C*x_);
P_est=(eye(n)-K*C)*P_;

== matlab function decoupling and rotation/decoupling /Embedded MATLAB Function ==
  data: pitch_cmd_comp output double; roll_cmd_comp output double; pitch_meas input double; thrust_comp output double; roll_meas input double; pitch_cmd input double; roll_cmd input double; thrust input double; m input double; g input double
function [pitch_cmd_comp, roll_cmd_comp, thrust_comp]  = fcn(pitch_meas, roll_meas, pitch_cmd, roll_cmd, thrust,m,g)
%#eml

thrust_comp=thrust/(cos(pitch_meas)*cos(roll_meas));

pitch_cmd_comp = m*g/thrust_comp*pitch_cmd;
roll_cmd_comp = m*g/thrust_comp*roll_cmd;

% pitch_cmd_comp=pitch_cmd;
% roll_cmd_comp=roll_cmd;
% pitch_cmd_comp = atan(Fx/(-thrust_comp));
% roll_cmd_comp = atan(Fy/(thrust_comp));

% pitch_cmd_comp = atan(Fx/(-thrust_comp));
% roll_cmd_comp = atan(Fy*cos(pitch_meas)/(thrust_comp));

== matlab function y states estimator/discrete kalman filter ==
  data: A input double; B input double; state_est output double; C input double; D input double; Q input double; R input double; u input double; y input double; P input double; state input double; P_est output double
function [state_est,P_est]  = fcn(A,B,C,D,Q,R, u, y, P, state)
%#eml

% Kalman filter according to Welch & Bishop, An Introduction to the Kalman
% Filter

n=size(A,1);

% Time update
x_=A*state+B*u;
P_=A*P*A'+Q;
  
% Measurement update
K=P_*C'*(C*P_*C'+R)^-1;
state_est=x_+K*(y-C*x_);
P_est=(eye(n)-K*C)*P_;

== matlab function z states estimator/discrete kalman filter ==
  data: A input double; B input double; state_est output double; C input double; D input double; Q input double; R input double; u input double; y input double; P input double; state input double; P_est output double
function [state_est,P_est]  = fcn(A,B,C,D,Q,R, u, y, P, state)
%#eml

% Kalman filter according to Welch & Bishop, An Introduction to the Kalman
% Filter

n=size(A,1);

% Time update
x_=A*state+B*u;
P_=A*P*A'+Q;
  
% Measurement update
K=P_*C'*(C*P_*C'+R)^-1;
state_est=x_+K*(y-C*x_);
P_est=(eye(n)-K*C)*P_;

== matlab function yaw states estimator/discrete kalman filter ==
  data: A input double; B input double; state_est output double; C input double; D input double; Q input double; R input double; u input double; y input double; P input double; state input double; P_est output double
function [state_est,P_est]  = fcn(A,B,C,D,Q,R, u, y, P, state)
%#eml

% Kalman filter according to Welch & Bishop, An Introduction to the Kalman
% Filter

n=size(A,1);

% Time update
x_=A*state+B*u;
P_=A*P*A'+Q;
  
% Measurement update
K=P_*C'*(C*P_*C'+R)^-1;
state_est=x_+K*(y-C*x_);
P_est=(eye(n)-K*C)*P_;

== matlab function decoupling and rotation/rotate_to_quat_frame/Embedded MATLAB Function ==
  data: yaw input double; pitch_rot output double; pitch_cmd input double; roll_cmd input double; roll_rot output double
function [pitch_rot,roll_rot] = fcn(yaw, pitch_cmd, roll_cmd)
% calculate the desired set angles, according to the derivation in chapter
% 5.1.3 ('Decoupled Position Control Approach')

sin_yaw=sin(yaw);
cos_yaw=cos(yaw);

R=[cos_yaw, sin_yaw; -sin_yaw, cos_yaw];

% take the inverse to rotate the commands back
temp=R'*[pitch_cmd;roll_cmd];
pitch_rot=temp(1);
roll_rot=temp(2);
